simulink model "sim_tase_2025_pos_ctrl"  (R2020a)
settings: Solver=ode4  StartTime=0.0  StopTime=30.0  FixedStep=0.01  RelTol=1e-3
values from neighbouring files (symbols this model uses):
  alfa_theta_obs = 100    [init_tase_2025_pos_ctrl.m]
  Aps = -diag([5, 5, 5])    [init_tase_2025_pos_ctrl.m]
  delta_p_i_0 = zeros(3, NF)    [init_tase_2025_pos_ctrl.m]
  delta_v_i_0 = zeros(3, NF)    [init_tase_2025_pos_ctrl.m]
  dp_aa_t = 0.2 * ones(3, 5) + ( 1.0 - 0.2 ) * rand(3, 5)    [init_tase_2025_pos_ctrl.m]
  dp_ff_t = [ 0.4 * ones(1, 5) + ( 1.0 - 0.4 ) * rand(1, 5);                      0.4 * ones(1, 5) + ( 1.0 - 0.4 ) * rand(1, 5);                      0.2 * ones(1, 5) + ( 0.6 - 0.2 ) * rand(1, 5) ]    [init_tase_2025_pos_ctrl.m]
  dp_phi_t = ( - pi / 2 ) * ones(3, 5) + ( pi / 2 - ( - pi / 2 ) ) * rand(3, 5)    [init_tase_2025_pos_ctrl.m]
  etai_0 = zeros(3,5)    [init_tase_2025_pos_ctrl.m]
  k_rho_1 = 10    [init_tase_2025_pos_ctrl.m]
  k_rho_2 = 10    [init_tase_2025_pos_ctrl.m]
  kai_1_t = 0.02    [init_tase_2025_pos_ctrl.m]
  kai_3_t = 0.1    [init_tase_2025_pos_ctrl.m]
  kp = 20    [init_tase_2025_pos_ctrl.m]
  ksii_0 = zeros(3,5)    [init_tase_2025_pos_ctrl.m]
  kv = 20    [init_tase_2025_pos_ctrl.m]
  l1v = diag([20; 20; 20])    [init_tase_2025_pos_ctrl.m]
  l2v = diag([30; 30; 30])    [init_tase_2025_pos_ctrl.m]
  mass_i = zeros(1,NF)    [init_tase_2025_pos_ctrl.m]
  Mii = diag([1;0;0;0;1])    [init_tase_2025_pos_ctrl.m]
  Phi_inv = inv( Aps ) * ( exp( Aps * tTs ) - eye(3) )    [init_tase_2025_pos_ctrl.m]
  pos0 = zeros(3, 1)    [init_tase_2025_pos_ctrl.m]
  PZ0 = P0(3)    [init_tase_2025_pos_ctrl.m]
  PZ1 = 10    [init_tase_2025_pos_ctrl.m]
  Qci_init = repmat([1;0;0;0],1,NF)    [init_tase_2025_pos_ctrl.m]
  R0 = 4    [init_tase_2025_pos_ctrl.m]
  R1 = 8    [init_tase_2025_pos_ctrl.m]
  Rx2 = 10    [init_tase_2025_pos_ctrl.m]
  Ry2 = 6    [init_tase_2025_pos_ctrl.m]
  Rz2 = 4    [init_tase_2025_pos_ctrl.m]
  T0 = 0    [init_tase_2025_pos_ctrl.m]
  T1 = tseq1    (= 10)    [init_tase_2025_pos_ctrl.m]
  T12 = tseq1 + tseq12    (= 20)    [init_tase_2025_pos_ctrl.m]
  T2 = tseq1 + tseq12 + tseq2    (= 30)    [init_tase_2025_pos_ctrl.m]
  theta0 = ( 2 / 5 ) * pi    (= 1.25663706144)    [init_tase_2025_pos_ctrl.m]
  theta_1 = 0    [init_tase_2025_pos_ctrl.m]
  theta_2 = 1    [init_tase_2025_pos_ctrl.m]
  TTb = 2    [init_tase_2025_pos_ctrl.m]
  tTs = 0.1    [init_tase_2025_pos_ctrl.m]
  vel0 = zeros(3, 1)    [init_tase_2025_pos_ctrl.m]
  Wij = [0,0,1,0,0;              0,0,1,1,0;              1,0,0,0,1;              0,1,1,0,0;              0,0,1,0,0]    [init_tase_2025_pos_ctrl.m]
  wp = 10    [init_tase_2025_pos_ctrl.m]
  X1 = 8    [init_tase_2025_pos_ctrl.m]
  X2 = 2    [init_tase_2025_pos_ctrl.m]
  X3 = 3    [init_tase_2025_pos_ctrl.m]
  Y1 = 10    [init_tase_2025_pos_ctrl.m]
  Y2 = 2    [init_tase_2025_pos_ctrl.m]
  Y3 = 4    [init_tase_2025_pos_ctrl.m]
  Z1 = 4    [init_tase_2025_pos_ctrl.m]
  Z2 = -6    [init_tase_2025_pos_ctrl.m]
  Z3 = 2    [init_tase_2025_pos_ctrl.m]
undefined symbols (not defined in the file or in its folder): cal_frac_squ, p_gamma1_pos, p_gamma1_vel, p_gamma2_pos, p_gamma2_vel, p_gamma_diff_1, p_gamma_diff_2_2, q_gamma1_pos, q_gamma1_vel, q_gamma2_pos, q_gamma2_vel, q_gamma_diff_1, q_gamma_diff_2_2
(part 2 of 4)

== matlab function sim_tase_2025_pos_ctrl/cal vel_diff_hat agent 3 ==
  data: k_rho_1 input; k_rho_2 input; TTb input; theta_1 input; theta_2 input; tsim input; ksi_diff_tilt_vec input; d_vel_diff_hat_3 output; sig_ksi_diff_tilt_gamma_1_vec input
function d_vel_diff_hat_3 = fcn(k_rho_1, k_rho_2, TTb, theta_1, theta_2, tsim, ksi_diff_tilt_vec, sig_ksi_diff_tilt_gamma_1_vec)
%%%% 计算高阶滑模微分器的速度估计
iiuav = 3;
if tsim < TTb
    theta = theta_1;
else
    theta = theta_2;
end
d_vel_diff_hat_3 = -theta * k_rho_1 * sign( ksi_diff_tilt_vec(:,iiuav) ) ...
                                    - ( 1 - theta ) * k_rho_2 * sig_ksi_diff_tilt_gamma_1_vec(:,iiuav);

== matlab function sim_tase_2025_pos_ctrl/desire formation position and velocity ==
  data: ksi0 input; eta0 input; delta_ksi_vec input; delta_eta_vec input; pos_i_des output; vel_i_des output
function [pos_i_des, vel_i_des] = fcn(ksi0, eta0, delta_ksi_vec, delta_eta_vec)
pos_i_des = zeros(3, 5);
vel_i_des = zeros(3, 5);
for iiuav = 1:5
    pos_i_des(:, iiuav) = ksi0(:) + delta_ksi_vec(:, iiuav);
    vel_i_des(:, iiuav) = eta0(:) + delta_eta_vec(:, iiuav);
end

== matlab function sim_tase_2025_pos_ctrl/cal vel_diff_hat agent 4 ==
  data: k_rho_1 input; k_rho_2 input; TTb input; theta_1 input; theta_2 input; tsim input; ksi_diff_tilt_vec input; d_vel_diff_hat_4 output; sig_ksi_diff_tilt_gamma_1_vec input
function d_vel_diff_hat_4 = fcn(k_rho_1, k_rho_2, TTb, theta_1, theta_2, tsim, ksi_diff_tilt_vec, sig_ksi_diff_tilt_gamma_1_vec)
%%%% 计算高阶滑模微分器的速度估计
iiuav = 4;
if tsim < TTb
    theta = theta_1;
else
    theta = theta_2;
end
d_vel_diff_hat_4 = -theta * k_rho_1 * sign( ksi_diff_tilt_vec(:,iiuav) ) ...
                                    - ( 1 - theta ) * k_rho_2 * sig_ksi_diff_tilt_gamma_1_vec(:,iiuav);

== matlab function sim_tase_2025_pos_ctrl/cal vel_diff_hat agent 5 ==
  data: k_rho_1 input; k_rho_2 input; TTb input; theta_1 input; theta_2 input; tsim input; ksi_diff_tilt_vec input; d_vel_diff_hat_5 output; sig_ksi_diff_tilt_gamma_1_vec input
function d_vel_diff_hat_5 = fcn(k_rho_1, k_rho_2, TTb, theta_1, theta_2, tsim, ksi_diff_tilt_vec, sig_ksi_diff_tilt_gamma_1_vec)
%%%% 计算高阶滑模微分器的速度估计
iiuav = 5;
if tsim < TTb
    theta = theta_1;
else
    theta = theta_2;
end
d_vel_diff_hat_5 = -theta * k_rho_1 * sign( ksi_diff_tilt_vec(:,iiuav) ) ...
                                    - ( 1 - theta ) * k_rho_2 * sig_ksi_diff_tilt_gamma_1_vec(:,iiuav);

== matlab function sim_tase_2025_pos_ctrl/combine vel_diff_hat ==
  data: vel_diff_hat_1 input; vel_diff_hat_vec output; vel_diff_hat_2 input; vel_diff_hat_3 input; vel_diff_hat_4 input; vel_diff_hat_5 input
function vel_diff_hat_vec = fcn(vel_diff_hat_1, vel_diff_hat_2, vel_diff_hat_3, vel_diff_hat_4, vel_diff_hat_5)
%%%% 合并绝对值幂次项
vel_diff_hat_vec = zeros(3,5);
vel_diff_hat_vec(:,1) = vel_diff_hat_1(:);
vel_diff_hat_vec(:,2) = vel_diff_hat_2(:);
vel_diff_hat_vec(:,3) = vel_diff_hat_3(:);
vel_diff_hat_vec(:,4) = vel_diff_hat_4(:);
vel_diff_hat_vec(:,5) = vel_diff_hat_5(:);

== matlab function sim_tase_2025_pos_ctrl/combine d_vel_diff_hat ==
  data: d_vel_diff_hat_1 input; d_vel_diff_hat_vec output; d_vel_diff_hat_2 input; d_vel_diff_hat_3 input; d_vel_diff_hat_4 input; d_vel_diff_hat_5 input
function d_vel_diff_hat_vec = fcn(d_vel_diff_hat_1, d_vel_diff_hat_2, d_vel_diff_hat_3, d_vel_diff_hat_4, d_vel_diff_hat_5)
%%%% 合并绝对值幂次项
d_vel_diff_hat_vec = zeros(3,5);
d_vel_diff_hat_vec(:,1) = d_vel_diff_hat_1(:);
d_vel_diff_hat_vec(:,2) = d_vel_diff_hat_2(:);
d_vel_diff_hat_vec(:,3) = d_vel_diff_hat_3(:);
d_vel_diff_hat_vec(:,4) = d_vel_diff_hat_4(:);
d_vel_diff_hat_vec(:,5) = d_vel_diff_hat_5(:);

== matlab function sim_tase_2025_pos_ctrl/cal pos_diff_hat agent 1 ==
  data: k_rho_1 input; k_rho_2 input; TTb input; theta_1 input; theta_2 input; tsim input; vel_diff_hat_vec input; d_pos_diff_hat_1 output; sig_ksi_diff_tilt_1_2_vec input; sig_ksi_diff_tilt_gamma_2_2_vec input
function d_pos_diff_hat_1 = fcn(k_rho_1, k_rho_2, TTb, theta_1, theta_2, tsim, ...
                                                            vel_diff_hat_vec, sig_ksi_diff_tilt_1_2_vec, sig_ksi_diff_tilt_gamma_2_2_vec)
%%%% 计算高阶滑模微分器的位置估计
iiuav = 1;
if tsim < TTb
    theta = theta_1;
else
    theta = theta_2;
end
d_pos_diff_hat_1 = vel_diff_hat_vec(:,iiuav) - theta * k_rho_1 * sig_ksi_diff_tilt_1_2_vec(:,iiuav) ...
                                    - ( 1 - theta ) * k_rho_2 * sig_ksi_diff_tilt_gamma_2_2_vec(:,iiuav);

== matlab function sim_tase_2025_pos_ctrl/cal pos_diff_hat agent 2 ==
  data: k_rho_1 input; k_rho_2 input; TTb input; theta_1 input; theta_2 input; tsim input; vel_diff_hat_vec input; d_pos_diff_hat_2 output; sig_ksi_diff_tilt_1_2_vec input; sig_ksi_diff_tilt_gamma_2_2_vec input
function d_pos_diff_hat_2 = fcn(k_rho_1, k_rho_2, TTb, theta_1, theta_2, tsim, ...
                                                            vel_diff_hat_vec, sig_ksi_diff_tilt_1_2_vec, sig_ksi_diff_tilt_gamma_2_2_vec)
%%%% 计算高阶滑模微分器的位置估计
iiuav = 2;
if tsim < TTb
    theta = theta_1;
else
    theta = theta_2;
end
d_pos_diff_hat_2 = vel_diff_hat_vec(:,iiuav) - theta * k_rho_1 * sig_ksi_diff_tilt_1_2_vec(:,iiuav) ...
                                    - ( 1 - theta ) * k_rho_2 * sig_ksi_diff_tilt_gamma_2_2_vec(:,iiuav);

== matlab function sim_tase_2025_pos_ctrl/cal pos_diff_hat agent 3 ==
  data: k_rho_1 input; k_rho_2 input; TTb input; theta_1 input; theta_2 input; tsim input; vel_diff_hat_vec input; d_pos_diff_hat_3 output; sig_ksi_diff_tilt_1_2_vec input; sig_ksi_diff_tilt_gamma_2_2_vec input
function d_pos_diff_hat_3 = fcn(k_rho_1, k_rho_2, TTb, theta_1, theta_2, tsim, ...
                                                            vel_diff_hat_vec, sig_ksi_diff_tilt_1_2_vec, sig_ksi_diff_tilt_gamma_2_2_vec)
%%%% 计算高阶滑模微分器的位置估计
iiuav = 3;
if tsim < TTb
    theta = theta_1;
else
    theta = theta_2;
end
d_pos_diff_hat_3 = vel_diff_hat_vec(:,iiuav) - theta * k_rho_1 * sig_ksi_diff_tilt_1_2_vec(:,iiuav) ...
                                    - ( 1 - theta ) * k_rho_2 * sig_ksi_diff_tilt_gamma_2_2_vec(:,iiuav);

== matlab function sim_tase_2025_pos_ctrl/cal pos_diff_hat agent 4 ==
  data: k_rho_1 input; k_rho_2 input; TTb input; theta_1 input; theta_2 input; tsim input; vel_diff_hat_vec input; d_pos_diff_hat_4 output; sig_ksi_diff_tilt_1_2_vec input; sig_ksi_diff_tilt_gamma_2_2_vec input
function d_pos_diff_hat_4 = fcn(k_rho_1, k_rho_2, TTb, theta_1, theta_2, tsim, ...
                                                            vel_diff_hat_vec, sig_ksi_diff_tilt_1_2_vec, sig_ksi_diff_tilt_gamma_2_2_vec)
%%%% 计算高阶滑模微分器的位置估计
iiuav = 4;
if tsim < TTb
    theta = theta_1;
else
    theta = theta_2;
end
d_pos_diff_hat_4 = vel_diff_hat_vec(:,iiuav) - theta * k_rho_1 * sig_ksi_diff_tilt_1_2_vec(:,iiuav) ...
                                    - ( 1 - theta ) * k_rho_2 * sig_ksi_diff_tilt_gamma_2_2_vec(:,iiuav);

== matlab function sim_tase_2025_pos_ctrl/generate translational disturbance agent 5 ==
  data: dp_aa_t input; dp_ff_t input; dp_phi_t input; dp_5 output; t input
function dp_5 = fcn(dp_aa_t, dp_ff_t, dp_phi_t, t)
%%%% 平移动力学方程中的扰动项设置
epsil_t = zeros(3, 1);

for kk = 1:5
    epsil_t = epsil_t + dp_aa_t(:, kk) .* sin( 2 * pi * dp_ff_t(:, kk) * t + dp_phi_t(:, kk) );
end

dp_5 = [ epsil_t(1) + 1.6 * sin( 0.2 * t ) + 2.0 * cos( 0.3 * t ) + 1.4 * sin( 0.5 * t ) ...
                + 4 * exp( -0.1 * t ) * sin( 0.5 * t ) + 3 / ( 1 + exp( -0.2 * ( t - 15 ) ) ); ...
                epsil_t(2) + 1.2 * sin( 0.1 * t ) + 3 * cos( 0.2 * t ) + 0.8 * sin( 0.4 * t ) ...
                + 2 * exp( -0.15 * t ) * cos( 0.6 * t ) + 3 / ( 1 + exp( -0.3 * ( t - 25 ) ) ); ...
                epsil_t(3) + 1.8 * sin( 0.1 * t ) + 1.6 * sin( 0.2 * t ) + 1.6 * cos( 0.3 * t ) ...
                + 4 * exp( -0.05 * t ) * sin( 0.4 * t + pi / 4 ) + 3 / ( 1 + exp( -0.5 * ( t - 20 ) ) ) ];

== matlab function sim_tase_2025_pos_ctrl/cal pos_diff_hat agent 5 ==
  data: k_rho_1 input; k_rho_2 input; TTb input; theta_1 input; theta_2 input; tsim input; vel_diff_hat_vec input; d_pos_diff_hat_5 output; sig_ksi_diff_tilt_1_2_vec input; sig_ksi_diff_tilt_gamma_2_2_vec input
function d_pos_diff_hat_5 = fcn(k_rho_1, k_rho_2, TTb, theta_1, theta_2, tsim, ...
                                                            vel_diff_hat_vec, sig_ksi_diff_tilt_1_2_vec, sig_ksi_diff_tilt_gamma_2_2_vec)
%%%% 计算高阶滑模微分器的位置估计
iiuav = 5;
if tsim < TTb
    theta = theta_1;
else
    theta = theta_2;
end
d_pos_diff_hat_5 = vel_diff_hat_vec(:,iiuav) - theta * k_rho_1 * sig_ksi_diff_tilt_1_2_vec(:,iiuav) ...
                                    - ( 1 - theta ) * k_rho_2 * sig_ksi_diff_tilt_gamma_2_2_vec(:,iiuav);

== matlab function sim_tase_2025_pos_ctrl/combine pos_diff_hat ==
  data: pos_diff_hat_1 input; pos_diff_hat_vec output; pos_diff_hat_2 input; pos_diff_hat_3 input; pos_diff_hat_4 input; pos_diff_hat_5 input
function pos_diff_hat_vec = fcn(pos_diff_hat_1, pos_diff_hat_2, pos_diff_hat_3, pos_diff_hat_4, pos_diff_hat_5)
%%%% 合并绝对值幂次项
pos_diff_hat_vec = zeros(3,5);
pos_diff_hat_vec(:,1) = pos_diff_hat_1(:);
pos_diff_hat_vec(:,2) = pos_diff_hat_2(:);
pos_diff_hat_vec(:,3) = pos_diff_hat_3(:);
pos_diff_hat_vec(:,4) = pos_diff_hat_4(:);
pos_diff_hat_vec(:,5) = pos_diff_hat_5(:);

== matlab function sim_tase_2025_pos_ctrl/choose eta_i agent 1 ==
  data: x input; y output
function y = fcn(x)
iiuav = 1;
y = x(:,iiuav);

== matlab function sim_tase_2025_pos_ctrl/choose eta_i agent 2 ==
  data: x input; y output
function y = fcn(x)
iiuav = 2;
y = x(:,iiuav);

== matlab function sim_tase_2025_pos_ctrl/choose eta_i agent 3 ==
  data: x input; y output
function y = fcn(x)
iiuav = 3;
y = x(:,iiuav);

== matlab function sim_tase_2025_pos_ctrl/choose eta_i agent 4 ==
  data: x input; y output
function y = fcn(x)
iiuav = 4;
y = x(:,iiuav);

== matlab function sim_tase_2025_pos_ctrl/choose eta_i agent 5 ==
  data: x input; y output
function y = fcn(x)
iiuav = 4;
y = x(:,iiuav);

== matlab function sim_tase_2025_pos_ctrl/choose ksi_i agent 1 ==
  data: x input; y output
function y = fcn(x)
iiuav = 1;
y = x(:,iiuav);

== matlab function sim_tase_2025_pos_ctrl/choose ksi_i agent 2 ==
  data: x input; y output
function y = fcn(x)
iiuav = 2;
y = x(:,iiuav);

== matlab function sim_tase_2025_pos_ctrl/choose ksi_i agent 3 ==
  data: x input; y output
function y = fcn(x)
iiuav = 3;
y = x(:,iiuav);

== matlab function sim_tase_2025_pos_ctrl/choose ksi_i agent 4 ==
  data: x input; y output
function y = fcn(x)
iiuav = 4;
y = x(:,iiuav);

== matlab function sim_tase_2025_pos_ctrl/choose ksi_i agent 5 ==
  data: x input; y output
function y = fcn(x)
iiuav = 4;
y = x(:,iiuav);

== matlab function sim_tase_2025_pos_ctrl/combine translational disturbance ==
  data: dp_vec output; dp_1 input; dp_2 input; dp_3 input; dp_4 input; dp_5 input
function dp_vec = fcn(dp_1, dp_2, dp_3, dp_4, dp_5)
%%%% 合并领导者编队跟踪误差结果
dp_vec = [dp_1(:), dp_2(:), dp_3(:), dp_4(:), dp_5(:)];

== matlab function sim_tase_2025_pos_ctrl/choose pos_diff_hat agent 1 ==
  data: x input; y output
function y = fcn(x)
iiuav = 1;
y = x(:,iiuav);

== matlab function sim_tase_2025_pos_ctrl/choose pos_diff_hat agent 2 ==
  data: x input; y output
function y = fcn(x)
iiuav = 2;
y = x(:,iiuav);

== matlab function sim_tase_2025_pos_ctrl/choose pos_diff_hat agent 3 ==
  data: x input; y output
function y = fcn(x)
iiuav = 3;
y = x(:,iiuav);

== matlab function sim_tase_2025_pos_ctrl/choose pos_diff_hat agent 4 ==
  data: x input; y output
function y = fcn(x)
iiuav = 4;
y = x(:,iiuav);

== matlab function sim_tase_2025_pos_ctrl/choose pos_diff_hat agent 5 ==
  data: x input; y output
function y = fcn(x)
iiuav = 4;
y = x(:,iiuav);

== matlab function sim_tase_2025_pos_ctrl/choose vel_diff_hat agent 1 ==
  data: x input; y output
function y = fcn(x)
iiuav = 1;
y = x(:,iiuav);

== matlab function sim_tase_2025_pos_ctrl/choose vel_diff_hat agent 2 ==
  data: x input; y output
function y = fcn(x)
iiuav = 2;
y = x(:,iiuav);

== matlab function sim_tase_2025_pos_ctrl/choose vel_diff_hat agent 3 ==
  data: x input; y output
function y = fcn(x)
iiuav = 3;
y = x(:,iiuav);

== matlab function sim_tase_2025_pos_ctrl/choose vel_diff_hat agent 4 ==
  data: x input; y output
function y = fcn(x)
iiuav = 4;
y = x(:,iiuav);

== matlab function sim_tase_2025_pos_ctrl/choose vel_diff_hat agent 5 ==
  data: x input; y output
function y = fcn(x)
iiuav = 4;
y = x(:,iiuav);

== matlab function sim_tase_2025_pos_ctrl/cal Rei ==
  data: Rei output; Qei input
function Rei = fcn(Qei)
%%%% 使用罗德里格公式由四元数Qei求解Rei
Rei = zeros(3,3,5);
for iuav = 1:5
    thetaei_tmp = Qei(1,iuav);
    qei_tmp = Qei(2:4,iuav);
    Rei(:,:,iuav) = ((thetaei_tmp^2) - (qei_tmp')*qei_tmp) * eye(3,3) ...
                            + 2 * qei_tmp * (qei_tmp') ...
                            - 2 * thetaei_tmp * cal_askew_mat(qei_tmp);
end

end

== matlab function sim_tase_2025_pos_ctrl/leader control input ==
  data: t input; u0 output; T1 input; T2 input; R0 input; R1 input; Rx2 input; Ry2 input; Rz2 input
function u0  = fcn(t, T1, T2, R0, R1, Rx2, Ry2, Rz2)
%%%% 给出领导者参考加速度控制输入
u0 = zeros(3, 1);

if t <= ( T1 + 1e-05 )
    u0(1, 1) = - ( 4 * pi * sin( ( 2 * pi * ( t - 0 ) ) / ( 0 - T1 ) ) * ( R0 - R1 ) ) / ( ( 0 - T1 ) ^ 2 ) ...
                        - ( 4 * ( pi ^ 2 ) * cos( ( 2 * pi * ( t - 0 ) ) / ( 0 - T1 ) ) ...
                        * ( R0 + ( ( R0 - R1 ) * ( t - 0 ) ) / ( 0 - T1 ) ) ) / ( ( 0 - T1 ) ^ 2 );
    u0(2, 1) = ( 4 * pi * cos( ( 2 * pi * ( t - 0 ) ) / ( 0 - T1 ) ) * ( R0 - R1 ) ) / ( ( 0 - T1 ) ^ 2 ) ...
                        - ( 4 * ( pi ^ 2 ) * sin( ( 2 * pi * ( t - 0 ) ) / ( 0 - T1 ) ) ...
                        * ( R0 + ( ( R0 - R1 ) * ( t - 0 ) ) / ( 0 - T1 ) ) ) / ( ( 0 - T1 ) ^ 2 );
    u0(3, 1) = 0;
else
    u0(1, 1) = ( 4 * Rx2 * ( pi ^ 2 ) * cos( ( 2 * pi * ( t - T1 ) ) / ( T1 - T2 ) ) ) / ( ( T1 - T2 ) ^ 2 );
    u0(2, 1) = - ( 16 * Ry2 * ( pi ^ 2 ) * sin( ( 4 * pi * ( t - T1 ) ) / ( T1 - T2 ) ) ) / ( ( T1 - T2 ) ^ 2 );
    u0(3, 1) = ( 16 * Rz2 * ( pi ^ 2 ) * sin( ( 4 * pi * ( t - T1 ) ) / ( T1 - T2 ) ) ) / ( ( T1 - T2 ) ^ 2 );
end

== matlab function sim_tase_2025_pos_ctrl/process velocity ==
  data: T0 input; T1 input; T2 input; PZ0 input; PZ1 input; R0 input; R1 input; Rx2 input; Ry2 input; Rz2 input; t input; V_init_out output
function V_init_out = fcn(T0, T1, T2, PZ0, PZ1, R0, R1, Rx2, Ry2, Rz2, t)
V_init_out = zeros(3, 1);
if t < T1 + 1e-05
    V_init_out(1, 1) = ( cos( ( 2 * pi * ( t - T0 ) ) / ( T0 - T1 ) ) * ( R0 - R1 ) ) / ( T0 - T1 ) ...
                                    - ( 2 * pi * sin( ( 2 * pi * ( t - T0 ) ) / ( T0 - T1 ) ) * ( R0 + ( ( R0 - R1 ) * ( t - T0 ) ) / ( T0 - T1 ) ) ) / ( T0 - T1 );
    V_init_out(2, 1) = ( sin( ( 2 * pi * ( t - T0 ) ) / ( T0 - T1 ) ) * ( R0 - R1 ) ) / ( T0 - T1 ) ...
                                    + ( 2 * pi * cos( ( 2 * pi * ( t - T0 ) ) / ( T0 - T1 ) ) * ( R0 + ( ( R0 - R1 ) * ( t - T0 ) ) / ( T0 - T1 ) ) ) / ( T0 - T1 );
    V_init_out(3, 1) = ( PZ0 - PZ1 ) / ( T0 - T1 );
else
    V_init_out(1, 1) = ( 2 * Rx2 * pi * sin( ( 2 * pi * ( t - T1 ) ) / ( T1 - T2 ) ) ) / ( T1 - T2 );
    V_init_out(2, 1) = ( 4 * Ry2 * pi * cos( ( 4 * pi * ( t - T1 ) ) / ( T1 - T2 ) ) ) / ( T1 - T2 );
    V_init_out(3, 1) = - ( 4 * Rz2 * pi * cos( ( 4 * pi * ( t - T1 ) ) / ( T1 - T2 ) ) ) / ( T1 - T2 );
end

== matlab function sim_tase_2025_pos_ctrl/cal formation tracking velocity errors ==
  data: wi0 input; err_eta_form_vec output; wij input; err_eta_vec input
function err_eta_form_vec = fcn(wi0, wij, err_eta_vec)
%%%% 计算编队跟踪误差
err_eta_form_vec = zeros(3,5);
for iiuav = 1:5
    err_eta_form_vec(:,iiuav) = wi0(iiuav, iiuav) * err_eta_vec(:,iiuav);
    for jjuav = 1:5
        err_eta_form_vec(:,iiuav) = err_eta_form_vec(:,iiuav) ...
                                                        + wij(iiuav, jjuav) * (err_eta_vec(:,iiuav) - err_eta_vec(:,jjuav));
    end
end

== matlab function sim_tase_2025_pos_ctrl/set desire formation configuration ==
  data: X1 input; X2 input; X3 input; Y1 input; Y2 input; Y3 input; Z1 input; Z2 input; Z3 input; theta0 input; kai_1_t input; kai_3_t input; T1 input; T12 input; t input; delta_ksi_vec output; delta_eta_vec output; d_delta_eta_vec output
function [delta_ksi_vec, delta_eta_vec, d_delta_eta_vec] = fcn(X1, X2, X3, Y1, Y2, Y3, Z1, Z2, Z3, ...
                                                                                                                theta0, kai_1_t, kai_3_t, T1, T12, t)
%%%% 计算跟随者期望速度分布式观测器误差
delta_ksi_vec = zeros(3, 5);
delta_eta_vec = zeros(3, 5);
d_delta_eta_vec = zeros(3, 5);
if t <= ( T1 + 1e-04 )
    exp_tmp = exp( -kai_1_t * t );
    delta_ksi_vec(:, 1) = [ X1 * cos( theta0 ) - X2 * exp_tmp; ...
                                            Y1 * sin( theta0 ) - Y2 * exp_tmp; ...
                                            Z1 - Z2 * exp_tmp ];
    delta_ksi_vec(:, 2) = [ - X1 * cos( theta0 ) + X2 * exp_tmp; ...
                                            Y1 * sin( theta0 ) - Y2 * exp_tmp; ...
                                            Z1 + Z2 * exp_tmp ];
    delta_ksi_vec(:, 3) = [ X1 - X2 * exp_tmp; ...
                                            Y2 * exp_tmp; ...
                                            ( 3 / 8 ) * Z1 + Z2 * exp_tmp ];
    delta_ksi_vec(:, 4) = [ - X1 * cos( theta0 ) + X2 * exp_tmp; ...
                                            - Y1 * sin( theta0 ) + Y2 * exp_tmp; ...
                                            Z1 + Z2 * exp_tmp ];
    delta_ksi_vec(:, 5) = [ X1 * cos( theta0 ) - X2 * exp_tmp; ...
                                            - Y1 * sin( theta0 ) + Y2 * exp_tmp; ...
                                            Z1 - Z2 * exp_tmp ];
    delta_eta_vec(:, 1) = [ kai_1_t * X2 * exp_tmp; kai_1_t * Y2 * exp_tmp; kai_1_t * Z2 * exp_tmp ];
    delta_eta_vec(:, 2) = [ - kai_1_t * X2 * exp_tmp; kai_1_t * Y2 * exp_tmp; - kai_1_t * Z2 * exp_tmp ];
    delta_eta_vec(:, 3) = [ kai_1_t * X2 * exp_tmp; - kai_1_t * Y2 * exp_tmp; - kai_1_t * Z2 * exp_tmp ];
    delta_eta_vec(:, 4) = [ - kai_1_t * X2 * exp_tmp; - kai_1_t * Y2 * exp_tmp; - kai_1_t * Z2 * exp_tmp ];
    delta_eta_vec(:, 5) = [ kai_1_t * X2 * exp_tmp; - kai_1_t * Y2 * exp_tmp; kai_1_t * Z2 * exp_tmp ];
    d_delta_eta_vec(:, 1) = [ - ( kai_1_t ^ 2 ) * X2 * exp_tmp; - ( kai_1_t ^ 2 ) * Y2 * exp_tmp; - ( kai_1_t ^ 2 ) * Z2 * exp_tmp ];
    d_delta_eta_vec(:, 2) = [ ( kai_1_t ^ 2 ) * X2 * exp_tmp; - ( kai_1_t ^ 2 ) * Y2 * exp_tmp; ( kai_1_t ^ 2 ) * Z2 * exp_tmp ];
    d_delta_eta_vec(:, 3) = [ - ( kai_1_t ^ 2 ) * X2 * exp_tmp; ( kai_1_t ^ 2 ) * Y2 * exp_tmp; ( kai_1_t ^ 2 ) * Z2 * exp_tmp ];
    d_delta_eta_vec(:, 4) = [ ( kai_1_t ^ 2 ) * X2 * exp_tmp; ( kai_1_t ^ 2 ) * Y2 * exp_tmp; ( kai_1_t ^ 2 ) * Z2 * exp_tmp ];
    d_delta_eta_vec(:, 5) = [ - ( kai_1_t ^ 2 ) * X2 * exp_tmp; ( kai_1_t ^ 2 ) * Y2 * exp_tmp; - ( kai_1_t ^ 2 ) * Z2 * exp_tmp ];
elseif t <= ( T12 + 1e-04 )
    delta_ksi_vec(:, 1) = [ X1 * cos( theta0 ) - X2; Y1 * sin( theta0 ) - Y2; Z1 - Z2 ];
    delta_ksi_vec(:, 2) = [ - X1 * cos( theta0 ) + X2; Y1 * sin( theta0 ) - Y2; Z1 + Z2 ];
    delta_ksi_vec(:, 3) = [ X1 - X2; 0; ( 3 / 8 ) * Z1 + Z2 ];
    delta_ksi_vec(:, 4) = [ - X1 * cos( theta0 ) + X2; - Y1 * sin( theta0 ) + Y2; Z1 + Z2 ];
    delta_ksi_vec(:, 5) = [ X1 * cos( theta0 ) - X2; - Y1 * sin( theta0 ) + Y2; Z1 - Z2 ];
else
    exp_tmp = 1 / ( 1 + exp( - kai_3_t * ( t - T12 - 5 ) ) );
    tmp_2 = exp( - kai_3_t * ( t - T12 - 5 ) ) / ( ( 1 + exp( - kai_3_t * ( t - T12 - 5 ) ) ) ^ 2 );
    delta_ksi_vec(:, 1) = [ X1 * cos( theta0 ) - X2 + X3 * exp_tmp; ...
                                            Y1 * sin( theta0 ) - Y2 + Y3 * exp_tmp; ...
                                            Z1 - Z2 + Z3 * exp_tmp ];
    delta_ksi_vec(:, 2) = [ - X1 * cos( theta0 ) + X2 - X3 * exp_tmp; ...
                                            Y1 * sin( theta0 ) - Y2 + Y3 * exp_tmp; ...
                                            Z1 + Z2 - Z3 * exp_tmp ];
    delta_ksi_vec(:, 3) = [ X1 - X2 + X3 * exp_tmp; ...
                                            - Y3 * exp_tmp; ...
                                            ( 3 / 8 ) * Z1 + Z2 - Z3 * exp_tmp ];
    delta_ksi_vec(:, 4) = [ - X1 * cos( theta0 ) + X2 - X3 * exp_tmp; ...
                                            - Y1 * sin( theta0 ) + Y2 - Y3 * exp_tmp; ...
                                            Z1 + Z2 - Z3 * exp_tmp ];
    delta_ksi_vec(:, 5) = [ X1 * cos( theta0 ) - X2 + X3 * exp_tmp; ...
                                            - Y1 * sin( theta0 ) + Y2 - Y3 * exp_tmp; ...
                                            Z1 - Z2 + Z3 * exp_tmp ];
    delta_eta_vec(:, 1) = [ kai_3_t * X3 * tmp_2; kai_3_t * Y3 * tmp_2; kai_3_t * Z3 * tmp_2 ];
    delta_eta_vec(:, 2) = [ - kai_3_t * X3 * tmp_2; kai_3_t * Y3 * tmp_2; kai_3_t * Z3 * tmp_2 ];
    delta_eta_vec(:, 3) = [ kai_3_t * X3 * tmp_2; - kai_3_t * Y3 * tmp_2; - kai_3_t * Z3 * tmp_2 ];
    delta_eta_vec(:, 4) = [ - kai_3_t * X3 * tmp_2; - kai_3_t * Y3 * tmp_2; - kai_3_t * Z3 * tmp_2 ];
    delta_eta_vec(:, 5) = [ kai_3_t * X3 * tmp_2; kai_3_t * Y3 * tmp_2; - kai_3_t * Z3 * tmp_2 ];
    d_delta_eta_vec(:, 1) = ( kai_3_t * ( 1 - exp( - kai_3_t * ( t - T12 - 5 ) ) ) * exp_tmp ) * delta_eta_vec(:, 1);
    d_delta_eta_vec(:, 2) = ( kai_3_t * ( 1 - exp( - kai_3_t * ( t - T12 - 5 ) ) ) * exp_tmp ) * delta_eta_vec(:, 2);
    d_delta_eta_vec(:, 3) = ( kai_3_t * ( 1 - exp( - kai_3_t * ( t - T12 - 5 ) ) ) * exp_tmp ) * delta_eta_vec(:, 3);
    d_delta_eta_vec(:, 4) = ( kai_3_t * ( 1 - exp( - kai_3_t * ( t - T12 - 5 ) ) ) * exp_tmp ) * delta_eta_vec(:, 4);
    d_delta_eta_vec(:, 5) = ( kai_3_t * ( 1 - exp( - kai_3_t * ( t - T12 - 5 ) ) ) * exp_tmp ) * delta_eta_vec(:, 5);
end

== matlab function sim_tase_2025_pos_ctrl/depart Re5 ==
  data: y output; x input
function y = fcn(x)
y = x(:,:,5);

end

== matlab function sim_tase_2025_pos_ctrl/depart Re1 ==
  data: y output; x input
function y = fcn(x)
y = x(:,:,1);

end

== matlab function sim_tase_2025_pos_ctrl/depart Re2 ==
  data: y output; x input
function y = fcn(x)
y = x(:,:,2);

end

== matlab function sim_tase_2025_pos_ctrl/depart Re3 ==
  data: y output; x input
function y = fcn(x)
y = x(:,:,3);

end

== matlab function sim_tase_2025_pos_ctrl/depart Re4 ==
  data: y output; x input
function y = fcn(x)
y = x(:,:,4);

end

== matlab function sim_tase_2025_pos_ctrl/cal Rci from ui ==
  data: Rci output; mi input; ui input
function Rci = fcn(mi, ui)
Rci = zeros(3,3,5);
for iiuav = 1:5
    Rci(:,:,iiuav) = cal_Rc_with_u(mi(iiuav), ui(:,iiuav));
end

end

== matlab function sim_tase_2025_pos_ctrl/cal abs 21 ==
  data: x input; y output
function y = fcn(x)
y = abs(x(:));

== matlab function sim_tase_2025_pos_ctrl/cal abs 22 ==
  data: x input; y output
function y = fcn(x)
y = abs(x(:));

== matlab function sim_tase_2025_pos_ctrl/choose ksi_diff_tilt ==
  data: x input; y output
function y = fcn(x)
iiuav = 1;
y = x(:,iiuav);

== matlab function sim_tase_2025_pos_ctrl/cal ui0 agent 2 ==
  data: kp input; ui0_2 output; kv input; u0 input; err_ksi_form_vec input; err_eta_form_vec input
function ui0_2 = fcn(kp, kv, u0, err_ksi_form_vec, err_eta_form_vec)
%%%% 计算标称控制输入ui0
iiuav = 2;
g0 = 9.80663;
e3 = [0;0;1];
ui0_2 = g0 * e3 + u0(:) - kp * err_ksi_form_vec(:,iiuav) ...
                - kv * err_eta_form_vec(:,iiuav);

== matlab function sim_tase_2025_pos_ctrl/choose ksi_diff_tilt 1 ==
  data: x input; y output
function y = fcn(x)
iiuav = 1;
y = x(:,iiuav);

== matlab function sim_tase_2025_pos_ctrl/trans to column20 ==
  data: x input; y output
function y = fcn(x)
y = x(:);

== matlab function sim_tase_2025_pos_ctrl/trans to column21 ==
  data: x input; y output
function y = fcn(x)
y = x(:);

== matlab function sim_tase_2025_pos_ctrl/cal dp_hat agent 1 ==
  data: Phi_inv input; mu_bTs_vec input; dp_hat_1 output
function dp_hat_1 = fcn(Phi_inv, mu_bTs_vec)
%%%% 计算扰动观测值dp_hat
iiuav = 1;
dp_hat_1 = -Phi_inv * mu_bTs_vec(:,iiuav);

== matlab function sim_tase_2025_pos_ctrl/combine dp_hat ==
  data: dp_hat_1 input; dp_hat_2 input; dp_hat_3 input; dp_hat_4 input; dp_hat_5 input; dp_hat_vec output
function dp_hat_vec  = fcn(dp_hat_1, dp_hat_2, dp_hat_3, dp_hat_4, dp_hat_5)
%%%% 合并扰动观测值dp_hat
dp_hat_vec = [dp_hat_1(:), dp_hat_2(:), dp_hat_3(:), dp_hat_4(:), dp_hat_5(:)];

== matlab function sim_tase_2025_pos_ctrl/cal ui0 agent 1 ==
  data: kp input; ui0_1 output; kv input; u0 input; err_ksi_form_vec input; err_eta_form_vec input
function ui0_1 = fcn(kp, kv, u0, err_ksi_form_vec, err_eta_form_vec)
%%%% 计算标称控制输入ui0
iiuav = 1;
g0 = 9.80663;
e3 = [0;0;1];
ui0_1 = g0 * e3 + u0(:) - kp * err_ksi_form_vec(:,iiuav) ...
                - kv * err_eta_form_vec(:,iiuav);

== matlab function sim_tase_2025_pos_ctrl/combine ui0 ==
  data: ui0_1 input; ui0_2 input; ui0_3 input; ui0_4 input; ui0_5 input; ui0 output
function ui0  = fcn(ui0_1, ui0_2, ui0_3, ui0_4, ui0_5)
%%%% 合并标称控制输入ui0
ui0 = [ui0_1(:), ui0_2(:), ui0_3(:), ui0_4(:), ui0_5(:)];

== matlab function sim_tase_2025_pos_ctrl/cal disturbance observation error dp_tilt ==
  data: dp_vec input; dp_tilt_vec output; dp_hat_vec input
function dp_tilt_vec = fcn(dp_vec, dp_hat_vec)
%%%% 计算扰动观测器估计误差dp_tilt
dp_tilt_vec = zeros(3,5);
for iiuav = 1:5
    dp_tilt_vec(:,iiuav) = dp_vec(:,iiuav) - dp_hat_vec(:,iiuav);
end

== matlab function sim_tase_2025_pos_ctrl/cal abs 41 ==
  data: x input; y output
function y = fcn(x)
y = abs(x(:));

== matlab function sim_tase_2025_pos_ctrl/cal abs 42 ==
  data: x input; y output
function y = fcn(x)
y = abs(x(:));

== matlab function sim_tase_2025_pos_ctrl/cal abs 43 ==
  data: x input; y output
function y = fcn(x)
y = abs(x(:));

== matlab function sim_tase_2025_pos_ctrl/cal abs 44 ==
  data: x input; y output
function y = fcn(x)
y = abs(x(:));

== matlab function sim_tase_2025_pos_ctrl/cal abs 45 ==
  data: x input; y output
function y = fcn(x)
y = abs(x(:));

== matlab function sim_tase_2025_pos_ctrl/cal abs 46 ==
  data: x input; y output
function y = fcn(x)
y = abs(x(:));

== matlab function sim_tase_2025_pos_ctrl/cal ui0 agent 3 ==
  data: kp input; ui0_3 output; kv input; u0 input; err_ksi_form_vec input; err_eta_form_vec input
function ui0_3 = fcn(kp, kv, u0, err_ksi_form_vec, err_eta_form_vec)
%%%% 计算标称控制输入ui0
iiuav = 3;
g0 = 9.80663;
e3 = [0;0;1];
ui0_3 = g0 * e3 + u0(:) - kp * err_ksi_form_vec(:,iiuav) ...
                - kv * err_eta_form_vec(:,iiuav);

== matlab function sim_tase_2025_pos_ctrl/cal abs 47 ==
  data: x input; y output
function y = fcn(x)
y = abs(x(:));

== matlab function sim_tase_2025_pos_ctrl/cal abs 48 ==
  data: x input; y output
function y = fcn(x)
y = abs(x(:));

== matlab function sim_tase_2025_pos_ctrl/cal abs 49 ==
  data: x input; y output
function y = fcn(x)
y = abs(x(:));

== matlab function sim_tase_2025_pos_ctrl/cal abs 50 ==
  data: x input; y output
function y = fcn(x)
y = abs(x(:));

== matlab function sim_tase_2025_pos_ctrl/cal abs 51 ==
  data: x input; y output
function y = fcn(x)
y = abs(x(:));

== matlab function sim_tase_2025_pos_ctrl/cal abs 52 ==
  data: x input; y output
function y = fcn(x)
y = abs(x(:));

== matlab function sim_tase_2025_pos_ctrl/cal abs 53 ==
  data: x input; y output
function y = fcn(x)
y = abs(x(:));

== matlab function sim_tase_2025_pos_ctrl/cal abs 54 ==
  data: x input; y output
function y = fcn(x)
y = abs(x(:));

== matlab function sim_tase_2025_pos_ctrl/cal abs 55 ==
  data: x input; y output
function y = fcn(x)
y = abs(x(:));

== matlab function sim_tase_2025_pos_ctrl/cal abs 56 ==
  data: x input; y output
function y = fcn(x)
y = abs(x(:));

== matlab function sim_tase_2025_pos_ctrl/cal abs 57 ==
  data: x input; y output
function y = fcn(x)
y = abs(x(:));

== matlab function sim_tase_2025_pos_ctrl/cal abs 58 ==
  data: x input; y output
function y = fcn(x)
y = abs(x(:));

== matlab function sim_tase_2025_pos_ctrl/cal abs 59 ==
  data: x input; y output
function y = fcn(x)
y = abs(x(:));

== matlab function sim_tase_2025_pos_ctrl/cal abs 60 ==
  data: x input; y output
function y = fcn(x)
y = abs(x(:));

== matlab function sim_tase_2025_pos_ctrl/cal lumped observation error agent 1 ==
  data: wij input; w0 input; ksi_d_est_vec input; ksi0 input; delta_ksi_vec input; eta_d_est_vec input; ksi_est_err_tilt_1 output; eta0 input; delta_eta_vec input; eta_est_err_tilt_1 output
function [ksi_est_err_tilt_1, eta_est_err_tilt_1]  = fcn(wij, w0, ksi_d_est_vec, ksi0, delta_ksi_vec, eta_d_est_vec, eta0, delta_eta_vec)
%%%% 计算跟随者期望速度分布式观测器误差
iiuav = 1;
ksi_est_err_tilt_1 = w0(iiuav, iiuav) * (ksi_d_est_vec(:,iiuav) - ksi0(:) - delta_ksi_vec(:,iiuav));
eta_est_err_tilt_1 = w0(iiuav, iiuav) * (eta_d_est_vec(:,iiuav) - eta0(:) - delta_eta_vec(:,iiuav));
for jjuav = 1:5
    ksi_est_err_tilt_1 = ksi_est_err_tilt_1 + ...
                                        wij(iiuav, jjuav) * ((ksi_d_est_vec(:,iiuav) - delta_ksi_vec(:,iiuav)) - (ksi_d_est_vec(:,jjuav) - delta_ksi_vec(:,jjuav)));
    eta_est_err_tilt_1 = eta_est_err_tilt_1 + ...
                                        wij(iiuav, jjuav) * ((eta_d_est_vec(:,iiuav) - delta_eta_vec(:,iiuav)) - (eta_d_est_vec(:,jjuav) - delta_eta_vec(:,jjuav)));
end

== matlab function sim_tase_2025_pos_ctrl/cal formation tracking position errors ==
  data: wi0 input; err_ksi_form_vec output; wij input; err_ksi_vec input
function err_ksi_form_vec = fcn(wi0, wij, err_ksi_vec)
%%%% 计算编队跟踪误差
err_ksi_form_vec = zeros(3,5);
for iiuav = 1:5
    err_ksi_form_vec(:,iiuav) = wi0(iiuav, iiuav) * err_ksi_vec(:,iiuav);
    for jjuav = 1:5
        err_ksi_form_vec(:,iiuav) = err_ksi_form_vec(:,iiuav) ...
                                                        + wij(iiuav, jjuav) * (err_ksi_vec(:,iiuav) - err_ksi_vec(:,jjuav));
    end
end

== matlab function sim_tase_2025_pos_ctrl/cal lumped observation error agent 2 ==
  data: wij input; w0 input; ksi_d_est_vec input; ksi0 input; delta_ksi_vec input; eta_d_est_vec input; ksi_est_err_tilt_2 output; eta0 input; delta_eta_vec input; eta_est_err_tilt_2 output
function [ksi_est_err_tilt_2, eta_est_err_tilt_2]  = fcn(wij, w0, ksi_d_est_vec, ksi0, delta_ksi_vec, eta_d_est_vec, eta0, delta_eta_vec)
%%%% 计算跟随者期望速度分布式观测器误差
iiuav = 2;
ksi_est_err_tilt_2 = w0(iiuav, iiuav) * (ksi_d_est_vec(:,iiuav) - ksi0(:) - delta_ksi_vec(:,iiuav));
eta_est_err_tilt_2 = w0(iiuav, iiuav) * (eta_d_est_vec(:,iiuav) - eta0(:) - delta_eta_vec(:,iiuav));
for jjuav = 1:5
    ksi_est_err_tilt_2 = ksi_est_err_tilt_2 + ...
                                        wij(iiuav, jjuav) * ((ksi_d_est_vec(:,iiuav) - delta_ksi_vec(:,iiuav)) - (ksi_d_est_vec(:,jjuav) - delta_ksi_vec(:,jjuav)));
    eta_est_err_tilt_2 = eta_est_err_tilt_2 + ...
                                        wij(iiuav, jjuav) * ((eta_d_est_vec(:,iiuav) - delta_eta_vec(:,iiuav)) - (eta_d_est_vec(:,jjuav) - delta_eta_vec(:,jjuav)));
end

== matlab function sim_tase_2025_pos_ctrl/cal lumped observation error agent 3 ==
  data: wij input; w0 input; ksi_d_est_vec input; ksi0 input; delta_ksi_vec input; eta_d_est_vec input; ksi_est_err_tilt_3 output; eta0 input; delta_eta_vec input; eta_est_err_tilt_3 output
function [ksi_est_err_tilt_3, eta_est_err_tilt_3]  = fcn(wij, w0, ksi_d_est_vec, ksi0, delta_ksi_vec, eta_d_est_vec, eta0, delta_eta_vec)
%%%% 计算跟随者期望速度分布式观测器误差
iiuav = 3;
ksi_est_err_tilt_3 = w0(iiuav, iiuav) * (ksi_d_est_vec(:,iiuav) - ksi0(:) - delta_ksi_vec(:,iiuav));
eta_est_err_tilt_3 = w0(iiuav, iiuav) * (eta_d_est_vec(:,iiuav) - eta0(:) - delta_eta_vec(:,iiuav));
for jjuav = 1:5
    ksi_est_err_tilt_3 = ksi_est_err_tilt_3 + ...
                                        wij(iiuav, jjuav) * ((ksi_d_est_vec(:,iiuav) - delta_ksi_vec(:,iiuav)) - (ksi_d_est_vec(:,jjuav) - delta_ksi_vec(:,jjuav)));
    eta_est_err_tilt_3 = eta_est_err_tilt_3 + ...
                                        wij(iiuav, jjuav) * ((eta_d_est_vec(:,iiuav) - delta_eta_vec(:,iiuav)) - (eta_d_est_vec(:,jjuav) - delta_eta_vec(:,jjuav)));
end

== matlab function sim_tase_2025_pos_ctrl/cal lumped observation error agent 4 ==
  data: wij input; w0 input; ksi_d_est_vec input; ksi0 input; delta_ksi_vec input; eta_d_est_vec input; ksi_est_err_tilt_4 output; eta0 input; delta_eta_vec input; eta_est_err_tilt_4 output
function [ksi_est_err_tilt_4, eta_est_err_tilt_4]  = fcn(wij, w0, ksi_d_est_vec, ksi0, delta_ksi_vec, eta_d_est_vec, eta0, delta_eta_vec)
%%%% 计算跟随者期望速度分布式观测器误差
iiuav = 4;
ksi_est_err_tilt_4 = w0(iiuav, iiuav) * (ksi_d_est_vec(:,iiuav) - ksi0(:) - delta_ksi_vec(:,iiuav));
eta_est_err_tilt_4 = w0(iiuav, iiuav) * (eta_d_est_vec(:,iiuav) - eta0(:) - delta_eta_vec(:,iiuav));
for jjuav = 1:5
    ksi_est_err_tilt_4 = ksi_est_err_tilt_4 + ...
                                        wij(iiuav, jjuav) * ((ksi_d_est_vec(:,iiuav) - delta_ksi_vec(:,iiuav)) - (ksi_d_est_vec(:,jjuav) - delta_ksi_vec(:,jjuav)));
    eta_est_err_tilt_4 = eta_est_err_tilt_4 + ...
                                        wij(iiuav, jjuav) * ((eta_d_est_vec(:,iiuav) - delta_eta_vec(:,iiuav)) - (eta_d_est_vec(:,jjuav) - delta_eta_vec(:,jjuav)));
end

== matlab function sim_tase_2025_pos_ctrl/cal lumped observation error agent 5 ==
  data: wij input; w0 input; ksi_d_est_vec input; ksi0 input; delta_ksi_vec input; eta_d_est_vec input; ksi_est_err_tilt_5 output; eta0 input; delta_eta_vec input; eta_est_err_tilt_5 output
function [ksi_est_err_tilt_5, eta_est_err_tilt_5]  = fcn(wij, w0, ksi_d_est_vec, ksi0, delta_ksi_vec, eta_d_est_vec, eta0, delta_eta_vec)
%%%% 计算跟随者期望速度分布式观测器误差
iiuav = 5;
ksi_est_err_tilt_5 = w0(iiuav, iiuav) * (ksi_d_est_vec(:,iiuav) - ksi0(:) - delta_ksi_vec(:,iiuav));
eta_est_err_tilt_5 = w0(iiuav, iiuav) * (eta_d_est_vec(:,iiuav) - eta0(:) - delta_eta_vec(:,iiuav));
for jjuav = 1:5
    ksi_est_err_tilt_5 = ksi_est_err_tilt_5 + ...
                                        wij(iiuav, jjuav) * ((ksi_d_est_vec(:,iiuav) - delta_ksi_vec(:,iiuav)) - (ksi_d_est_vec(:,jjuav) - delta_ksi_vec(:,jjuav)));
    eta_est_err_tilt_5 = eta_est_err_tilt_5 + ...
                                        wij(iiuav, jjuav) * ((eta_d_est_vec(:,iiuav) - delta_eta_vec(:,iiuav)) - (eta_d_est_vec(:,jjuav) - delta_eta_vec(:,jjuav)));
end

== matlab function sim_tase_2025_pos_ctrl/cal position estimate error ==
  data: ksi_d_est_vec input; ksi_est_err output; ksi0 input; delta_ksi_vec input
function ksi_est_err  = fcn(ksi_d_est_vec, ksi0, delta_ksi_vec)
%%%% 计算跟随者期望位置分布式观测器误差
ksi_est_err = ksi_d_est_vec - repmat(ksi0, 1, 5) - delta_ksi_vec;

== matlab function sim_tase_2025_pos_ctrl/cal theta_eta_est_err_tilt agent 1 ==
  data: alfa_theta input; eta_est_err_squ_1_node_1 input; theta_eta_est_err_tilt_1_1 output; eta_est_err_squ_2_node_1 input; eta_est_err_tilt_vec input; theta_eta_est_err_tilt_2_1 output
function [theta_eta_est_err_tilt_1_1, theta_eta_est_err_tilt_2_1] = fcn(alfa_theta, eta_est_err_squ_1_node_1, eta_est_err_squ_2_node_1, eta_est_err_tilt_vec)
%%%% 计算平滑递增函数
iiuav = 1;
theta_eta_est_err_tilt_1_1 = eta_est_err_squ_1_node_1(:) .* ( -1 + 2 ./ ( 1 + exp( -alfa_theta .* eta_est_err_tilt_vec(:,iiuav) ) ) );
theta_eta_est_err_tilt_2_1 = eta_est_err_squ_2_node_1(:) .* ( -1 + 2 ./ ( 1 + exp( -alfa_theta .* eta_est_err_tilt_vec(:,iiuav) ) ) );

== matlab function sim_tase_2025_pos_ctrl/cal theta_eta_est_err_tilt agent 2 ==
  data: alfa_theta input; eta_est_err_squ_1_node_2 input; theta_eta_est_err_tilt_1_2 output; eta_est_err_squ_2_node_2 input; eta_est_err_tilt_vec input; theta_eta_est_err_tilt_2_2 output
function [theta_eta_est_err_tilt_1_2, theta_eta_est_err_tilt_2_2] = fcn(alfa_theta, eta_est_err_squ_1_node_2, eta_est_err_squ_2_node_2, eta_est_err_tilt_vec)
%%%% 计算平滑递增函数
iiuav = 2;
theta_eta_est_err_tilt_1_2 = eta_est_err_squ_1_node_2(:) .* ( -1 + 2 ./ ( 1 + exp( -alfa_theta .* eta_est_err_tilt_vec(:,iiuav) ) ) );
theta_eta_est_err_tilt_2_2 = eta_est_err_squ_2_node_2(:) .* ( -1 + 2 ./ ( 1 + exp( -alfa_theta .* eta_est_err_tilt_vec(:,iiuav) ) ) );

== matlab function sim_tase_2025_pos_ctrl/cal ui0 agent 4 ==
  data: kp input; ui0_4 output; kv input; u0 input; err_ksi_form_vec input; err_eta_form_vec input
function ui0_4 = fcn(kp, kv, u0, err_ksi_form_vec, err_eta_form_vec)
%%%% 计算标称控制输入ui0
iiuav = 4;
g0 = 9.80663;
e3 = [0;0;1];
ui0_4 = g0 * e3 + u0(:) - kp * err_ksi_form_vec(:,iiuav) ...
                - kv * err_eta_form_vec(:,iiuav);

== matlab function sim_tase_2025_pos_ctrl/cal theta_eta_est_err_tilt agent 3 ==
  data: alfa_theta input; eta_est_err_squ_1_node_3 input; theta_eta_est_err_tilt_1_3 output; eta_est_err_squ_2_node_3 input; eta_est_err_tilt_vec input; theta_eta_est_err_tilt_2_3 output
function [theta_eta_est_err_tilt_1_3, theta_eta_est_err_tilt_2_3] = fcn(alfa_theta, eta_est_err_squ_1_node_3, eta_est_err_squ_2_node_3, eta_est_err_tilt_vec)
%%%% 计算平滑递增函数
iiuav = 3;
theta_eta_est_err_tilt_1_3 = eta_est_err_squ_1_node_3(:) .* ( -1 + 2 ./ ( 1 + exp( -alfa_theta .* eta_est_err_tilt_vec(:,iiuav) ) ) );
theta_eta_est_err_tilt_2_3 = eta_est_err_squ_2_node_3(:) .* ( -1 + 2 ./ ( 1 + exp( -alfa_theta .* eta_est_err_tilt_vec(:,iiuav) ) ) );

== matlab function sim_tase_2025_pos_ctrl/cal theta_eta_est_err_tilt agent 4 ==
  data: alfa_theta input; eta_est_err_squ_1_node_4 input; theta_eta_est_err_tilt_1_4 output; eta_est_err_squ_2_node_4 input; eta_est_err_tilt_vec input; theta_eta_est_err_tilt_2_4 output
function [theta_eta_est_err_tilt_1_4, theta_eta_est_err_tilt_2_4] = fcn(alfa_theta, eta_est_err_squ_1_node_4, eta_est_err_squ_2_node_4, eta_est_err_tilt_vec)
%%%% 计算平滑递增函数
iiuav = 4;
theta_eta_est_err_tilt_1_4 = eta_est_err_squ_1_node_4(:) .* ( -1 + 2 ./ ( 1 + exp( -alfa_theta .* eta_est_err_tilt_vec(:,iiuav) ) ) );
theta_eta_est_err_tilt_2_4 = eta_est_err_squ_2_node_4(:) .* ( -1 + 2 ./ ( 1 + exp( -alfa_theta .* eta_est_err_tilt_vec(:,iiuav) ) ) );

== matlab function sim_tase_2025_pos_ctrl/cal theta_eta_est_err_tilt agent 5 ==
  data: alfa_theta input; eta_est_err_squ_1_node_5 input; theta_eta_est_err_tilt_1_5 output; eta_est_err_squ_2_node_5 input; eta_est_err_tilt_vec input; theta_eta_est_err_tilt_2_5 output
function [theta_eta_est_err_tilt_1_5, theta_eta_est_err_tilt_2_5] = fcn(alfa_theta, eta_est_err_squ_1_node_5, eta_est_err_squ_2_node_5, eta_est_err_tilt_vec)
%%%% 计算平滑递增函数
iiuav = 5;
theta_eta_est_err_tilt_1_5 = eta_est_err_squ_1_node_5(:) .* ( -1 + 2 ./ ( 1 + exp( -alfa_theta .* eta_est_err_tilt_vec(:,iiuav) ) ) );
theta_eta_est_err_tilt_2_5 = eta_est_err_squ_2_node_5(:) .* ( -1 + 2 ./ ( 1 + exp( -alfa_theta .* eta_est_err_tilt_vec(:,iiuav) ) ) );

== matlab function sim_tase_2025_pos_ctrl/cal theta_ksi_est_err_tilt agent 1 ==
  data: alfa_theta input; ksi_est_err_squ_1_node_1 input; theta_ksi_est_err_tilt_1_1 output; ksi_est_err_squ_2_node_1 input; ksi_est_err_tilt_vec input; theta_ksi_est_err_tilt_2_1 output
function [theta_ksi_est_err_tilt_1_1, theta_ksi_est_err_tilt_2_1] = fcn(alfa_theta, ksi_est_err_squ_1_node_1, ksi_est_err_squ_2_node_1, ksi_est_err_tilt_vec)
%%%% 计算平滑递增函数
iiuav = 1;
theta_ksi_est_err_tilt_1_1 = ksi_est_err_squ_1_node_1(:) .* ( -1 + 2 ./ ( 1 + exp( -alfa_theta .* ksi_est_err_tilt_vec(:,iiuav) ) ) );
theta_ksi_est_err_tilt_2_1 = ksi_est_err_squ_2_node_1(:) .* ( -1 + 2 ./ ( 1 + exp( -alfa_theta .* ksi_est_err_tilt_vec(:,iiuav) ) ) );

== matlab function sim_tase_2025_pos_ctrl/cal theta_ksi_est_err_tilt agent 2 ==
  data: alfa_theta input; ksi_est_err_squ_1_node_2 input; theta_ksi_est_err_tilt_1_2 output; ksi_est_err_squ_2_node_2 input; ksi_est_err_tilt_vec input; theta_ksi_est_err_tilt_2_2 output
function [theta_ksi_est_err_tilt_1_2, theta_ksi_est_err_tilt_2_2] = fcn(alfa_theta, ksi_est_err_squ_1_node_2, ksi_est_err_squ_2_node_2, ksi_est_err_tilt_vec)
%%%% 计算平滑递增函数
iiuav = 2;
theta_ksi_est_err_tilt_1_2 = ksi_est_err_squ_1_node_2(:) .* ( -1 + 2 ./ ( 1 + exp( -alfa_theta .* ksi_est_err_tilt_vec(:,iiuav) ) ) );
theta_ksi_est_err_tilt_2_2 = ksi_est_err_squ_2_node_2(:) .* ( -1 + 2 ./ ( 1 + exp( -alfa_theta .* ksi_est_err_tilt_vec(:,iiuav) ) ) );

== matlab function sim_tase_2025_pos_ctrl/cal theta_ksi_est_err_tilt agent 3 ==
  data: alfa_theta input; ksi_est_err_squ_1_node_3 input; theta_ksi_est_err_tilt_1_3 output; ksi_est_err_squ_2_node_3 input; ksi_est_err_tilt_vec input; theta_ksi_est_err_tilt_2_3 output
function [theta_ksi_est_err_tilt_1_3, theta_ksi_est_err_tilt_2_3] = fcn(alfa_theta, ksi_est_err_squ_1_node_3, ksi_est_err_squ_2_node_3, ksi_est_err_tilt_vec)
%%%% 计算平滑递增函数
iiuav = 3;
theta_ksi_est_err_tilt_1_3 = ksi_est_err_squ_1_node_3(:) .* ( -1 + 2 ./ ( 1 + exp( -alfa_theta .* ksi_est_err_tilt_vec(:,iiuav) ) ) );
theta_ksi_est_err_tilt_2_3 = ksi_est_err_squ_2_node_3(:) .* ( -1 + 2 ./ ( 1 + exp( -alfa_theta .* ksi_est_err_tilt_vec(:,iiuav) ) ) );

== matlab function sim_tase_2025_pos_ctrl/cal theta_ksi_est_err_tilt agent 4 ==
  data: alfa_theta input; ksi_est_err_squ_1_node_4 input; theta_ksi_est_err_tilt_1_4 output; ksi_est_err_squ_2_node_4 input; ksi_est_err_tilt_vec input; theta_ksi_est_err_tilt_2_4 output
function [theta_ksi_est_err_tilt_1_4, theta_ksi_est_err_tilt_2_4] = fcn(alfa_theta, ksi_est_err_squ_1_node_4, ksi_est_err_squ_2_node_4, ksi_est_err_tilt_vec)
%%%% 计算平滑递增函数
iiuav = 4;
theta_ksi_est_err_tilt_1_4 = ksi_est_err_squ_1_node_4(:) .* ( -1 + 2 ./ ( 1 + exp( -alfa_theta .* ksi_est_err_tilt_vec(:,iiuav) ) ) );
theta_ksi_est_err_tilt_2_4 = ksi_est_err_squ_2_node_4(:) .* ( -1 + 2 ./ ( 1 + exp( -alfa_theta .* ksi_est_err_tilt_vec(:,iiuav) ) ) );

== matlab function sim_tase_2025_pos_ctrl/cal theta_ksi_est_err_tilt agent 5 ==
  data: alfa_theta input; ksi_est_err_squ_1_node_5 input; theta_ksi_est_err_tilt_1_5 output; ksi_est_err_squ_2_node_5 input; ksi_est_err_tilt_vec input; theta_ksi_est_err_tilt_2_5 output
function [theta_ksi_est_err_tilt_1_5, theta_ksi_est_err_tilt_2_5] = fcn(alfa_theta, ksi_est_err_squ_1_node_5, ksi_est_err_squ_2_node_5, ksi_est_err_tilt_vec)
%%%% 计算平滑递增函数
iiuav = 5;
theta_ksi_est_err_tilt_1_5 = ksi_est_err_squ_1_node_5(:) .* ( -1 + 2 ./ ( 1 + exp( -alfa_theta .* ksi_est_err_tilt_vec(:,iiuav) ) ) );
theta_ksi_est_err_tilt_2_5 = ksi_est_err_squ_2_node_5(:) .* ( -1 + 2 ./ ( 1 + exp( -alfa_theta .* ksi_est_err_tilt_vec(:,iiuav) ) ) );

== matlab function sim_tase_2025_pos_ctrl/cal velocity estimate error ==
  data: eta_d_est_vec input; eta_est_err output; eta0 input; delta_eta_vec input
function eta_est_err  = fcn(eta_d_est_vec, eta0, delta_eta_vec)
%%%% 计算跟随者期望速度分布式观测器误差
eta_est_err = eta_d_est_vec - repmat(eta0, 1, 5) - delta_eta_vec;

== matlab function sim_tase_2025_pos_ctrl/choose eta_est_err_tilt 1 ==
  data: x input; y output
function y = fcn(x)
iiuav = 1;
y = x(:,iiuav);

== matlab function sim_tase_2025_pos_ctrl/cal ui0 agent 5 ==
  data: kp input; ui0_5 output; kv input; u0 input; err_ksi_form_vec input; err_eta_form_vec input
function ui0_5 = fcn(kp, kv, u0, err_ksi_form_vec, err_eta_form_vec)
%%%% 计算标称控制输入ui0
iiuav = 5;
g0 = 9.80663;
e3 = [0;0;1];
ui0_5 = g0 * e3 + u0(:) - kp * err_ksi_form_vec(:,iiuav) ...
                - kv * err_eta_form_vec(:,iiuav);

== matlab function sim_tase_2025_pos_ctrl/choose eta_est_err_tilt 10 ==
  data: x input; y output
function y = fcn(x)
iiuav = 5;
y = x(:,iiuav);

== matlab function sim_tase_2025_pos_ctrl/choose eta_est_err_tilt 11 ==
  data: x input; y output
function y = fcn(x)
iiuav = 1;
y = x(:,iiuav);

== matlab function sim_tase_2025_pos_ctrl/choose eta_est_err_tilt 12 ==
  data: x input; y output
function y = fcn(x)
iiuav = 5;
y = x(:,iiuav);

== matlab function sim_tase_2025_pos_ctrl/choose eta_est_err_tilt 13 ==
  data: x input; y output
function y = fcn(x)
iiuav = 1;
y = x(:,iiuav);

== matlab function sim_tase_2025_pos_ctrl/choose eta_est_err_tilt 14 ==
  data: x input; y output
function y = fcn(x)
iiuav = 2;
y = x(:,iiuav);

== matlab function sim_tase_2025_pos_ctrl/choose eta_est_err_tilt 15 ==
  data: x input; y output
function y = fcn(x)
iiuav = 2;
y = x(:,iiuav);

== matlab function sim_tase_2025_pos_ctrl/choose eta_est_err_tilt 16 ==
  data: x input; y output
function y = fcn(x)
iiuav = 3;
y = x(:,iiuav);

== matlab function sim_tase_2025_pos_ctrl/choose eta_est_err_tilt 17 ==
  data: x input; y output
function y = fcn(x)
iiuav = 3;
y = x(:,iiuav);

== matlab function sim_tase_2025_pos_ctrl/choose eta_est_err_tilt 18 ==
  data: x input; y output
function y = fcn(x)
iiuav = 4;
y = x(:,iiuav);

== matlab function sim_tase_2025_pos_ctrl/choose eta_est_err_tilt 19 ==
  data: x input; y output
function y = fcn(x)
iiuav = 4;
y = x(:,iiuav);

== matlab function sim_tase_2025_pos_ctrl/choose eta_est_err_tilt 2 ==
  data: x input; y output
function y = fcn(x)
iiuav = 1;
y = x(:,iiuav);

== matlab function sim_tase_2025_pos_ctrl/choose eta_est_err_tilt 20 ==
  data: x input; y output
function y = fcn(x)
iiuav = 5;
y = x(:,iiuav);

== matlab function sim_tase_2025_pos_ctrl/choose eta_est_err_tilt 3 ==
  data: x input; y output
function y = fcn(x)
iiuav = 2;
y = x(:,iiuav);

== matlab function sim_tase_2025_pos_ctrl/choose eta_est_err_tilt 4 ==
  data: x input; y output
function y = fcn(x)
iiuav = 2;
y = x(:,iiuav);

== matlab function sim_tase_2025_pos_ctrl/choose eta_est_err_tilt 5 ==
  data: x input; y output
function y = fcn(x)
iiuav = 3;
y = x(:,iiuav);

== matlab function sim_tase_2025_pos_ctrl/choose eta_est_err_tilt 6 ==
  data: x input; y output
function y = fcn(x)
iiuav = 3;
y = x(:,iiuav);

== matlab function sim_tase_2025_pos_ctrl/update vl_hat agent 1 ==
  data: Aps input; d_vl_hat_1 output; ui0 input; ui1 input; dp_hat_vec input; vli_tilt_vec input
function d_vl_hat_1 = fcn(Aps, ui0, ui1, dp_hat_vec, vli_tilt_vec)
%%%% 更新状态预测器
iiuav = 1;
g0 = 9.80663;
e3 = [0;0;1];
d_vl_hat_1 = -g0 * e3 + ui0(:,iiuav) + dp_hat_vec(:,iiuav) ...
                        + ui1(:,iiuav) + Aps * vli_tilt_vec(:,iiuav);

== matlab function sim_tase_2025_pos_ctrl/choose eta_est_err_tilt 7 ==
  data: x input; y output
function y = fcn(x)
iiuav = 4;
y = x(:,iiuav);

== matlab function sim_tase_2025_pos_ctrl/choose eta_est_err_tilt 8 ==
  data: x input; y output
function y = fcn(x)
iiuav = 4;
y = x(:,iiuav);

== matlab function sim_tase_2025_pos_ctrl/choose eta_est_err_tilt 9 ==
  data: x input; y output
function y = fcn(x)
iiuav = 5;
y = x(:,iiuav);

== matlab function sim_tase_2025_pos_ctrl/combine follower desire velocity estimaters ==
  data: eta_d_est_1 input; eta_d_est_vec output; eta_d_est_2 input; eta_d_est_3 input; eta_d_est_4 input; eta_d_est_5 input
function eta_d_est_vec = fcn(eta_d_est_1, eta_d_est_2, eta_d_est_3, eta_d_est_4, eta_d_est_5)
%%%% 合并领导者位置观测器输出结果
eta_d_est_vec = [eta_d_est_1(:), eta_d_est_2(:), eta_d_est_3(:), eta_d_est_4(:), eta_d_est_5(:)];
